simulink model "RegolazioneDinamicaSistemaNonLineare_mdl"  (Simulink 7.2)
settings: Solver=ode45  StartTime=0.0  StopTime=30  RelTol=1e-3
values from neighbouring files (symbols this model uses):
  b = 0.0575    [TSC150918ProvaMatlab.m]
  C1 = [1 -1 0 0]    [TSC150918ProvaMatlab.m]
  d = 2.5185    [TSC150918ProvaMatlab.m]
  g = 9.81    [TSC150918ProvaMatlab.m]
  j = 0.2156    [TSC150918ProvaMatlab.m]
  k = 200    [TSC150918ProvaMatlab.m]
  l = 0.5    [TSC150918ProvaMatlab.m]
  L = - acker(A',C1',Po)'    [TSC150918ProvaMatlab.m]
  m = 0.15    [TSC150918ProvaMatlab.m]
  taue = 0.2    [TSC150918ProvaMatlab.m]
  X0 = Xe + Dx0    [TSC150918ProvaMatlab.m]
undefined symbols (not defined in the file or in its folder): A, B, K
settings Model: Creator=lbiagiotti  LastModifiedBy=lbiagiotti

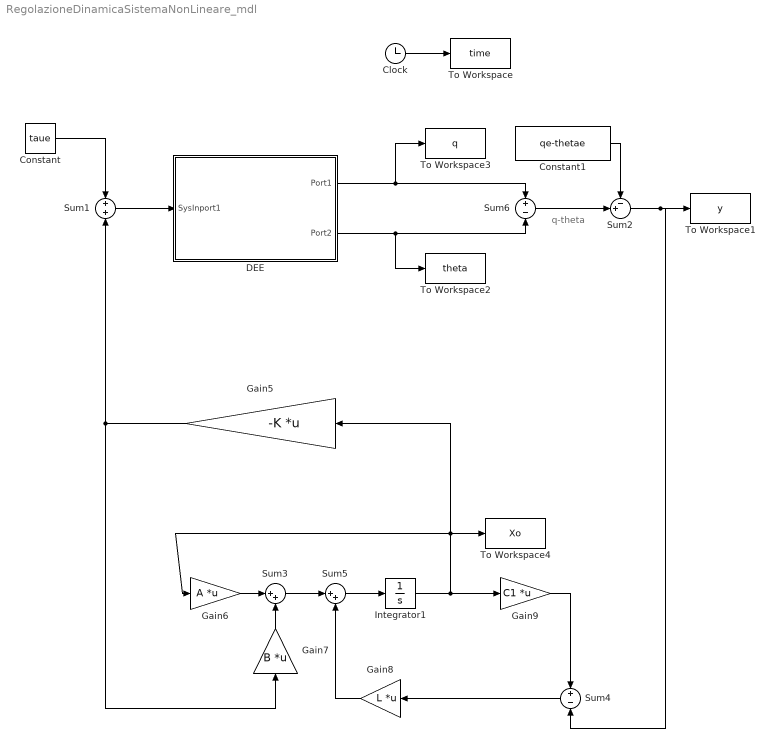
== system RegolazioneDinamicaSistemaNonLineare_mdl ==
  note: q-theta
  Clock : Clock
      settings: Decimation=10
  Constant : Constant  Value=taue  OutDataType=sfix(16)  OutScaling=2^0
  Constant1 : Constant  Value=qe-thetae  OutDataType=sfix(16)  OutScaling=2^0
  DEE : Subsystem
      settings: OpenFcn=diffeqed
      mask Type: Differential Equation Editor (DEE)
      mask Display: disp('Differential Equation\n Editor')
  Gain5 : Gain  Orientation=left  Gain=-K  Multiplication=Matrix(K*u)  ParameterDataType=sfix(16)  ParameterScaling=2^0  OutDataType=sfix(16)  OutScaling=2^0
  Gain6 : Gain  Gain=A  Multiplication=Matrix(K*u)  ParameterDataType=sfix(16)  ParameterScaling=2^0  OutDataType=sfix(16)  OutScaling=2^0
  Gain7 : Gain  Orientation=up  Gain=B  Multiplication=Matrix(K*u)  ParameterDataType=sfix(16)  ParameterScaling=2^0  OutDataType=sfix(16)  OutScaling=2^0
  Gain8 : Gain  Orientation=left  Gain=L  Multiplication=Matrix(K*u)  ParameterDataType=sfix(16)  ParameterScaling=2^0  OutDataType=sfix(16)  OutScaling=2^0
  Gain9 : Gain  Gain=C1  Multiplication=Matrix(K*u)  ParameterDataType=sfix(16)  ParameterScaling=2^0  OutDataType=sfix(16)  OutScaling=2^0
  Integrator1 : Integrator  InitialCondition=[0 0 0 0]
  Sum1 : Sum  OutDataType=sfix(16)  OutScaling=2^0
  Sum2 : Sum  Inputs=-+|  OutDataType=sfix(16)  OutScaling=2^0
  Sum3 : Sum  Inputs=|++  OutDataType=sfix(16)  OutScaling=2^0
  Sum4 : Sum  Orientation=left  Inputs=+-  OutDataType=sfix(16)  OutScaling=2^0
  Sum5 : Sum  Inputs=|++  OutDataType=sfix(16)  OutScaling=2^0
  Sum6 : Sum  Inputs=+-  OutDataType=sfix(16)  OutScaling=2^0
  To Workspace : ToWorkspace  VariableName=time  SampleTime=-1  SaveFormat=Array
  To Workspace1 : ToWorkspace  VariableName=y  SampleTime=-1  SaveFormat=Array
  To Workspace2 : ToWorkspace  VariableName=theta  SampleTime=-1  SaveFormat=Array
  To Workspace3 : ToWorkspace  VariableName=q  SampleTime=-1  SaveFormat=Array
  To Workspace4 : ToWorkspace  VariableName=Xo  SampleTime=-1  SaveFormat=Array
  wires:
  Clock/1 -> To Workspace/1
  Gain5/1 -> Gain7/1, Sum1/2
  Gain6/1 -> Sum3/1
  Integrator1/1 -> Gain9/1, Gain6/1, To Workspace4/1, Gain5/1
  Gain7/1 -> Sum3/2
  Sum4/1 -> Gain8/1
  Gain8/1 -> Sum5/2
  Sum3/1 -> Sum5/1
  Sum5/1 -> Integrator1/1
  Gain9/1 -> Sum4/1
  Sum1/1 -> DEE/1(SysInport1)
  Constant/1 -> Sum1/1
  Sum2/1 -> To Workspace1/1, Sum4/2
  Constant1/1 -> Sum2/1
  DEE/1(Port1) -> Sum6/1, To Workspace3/1
  DEE/2(Port2) -> Sum6/2, To Workspace2/1
  Sum6/1 -> Sum2/2

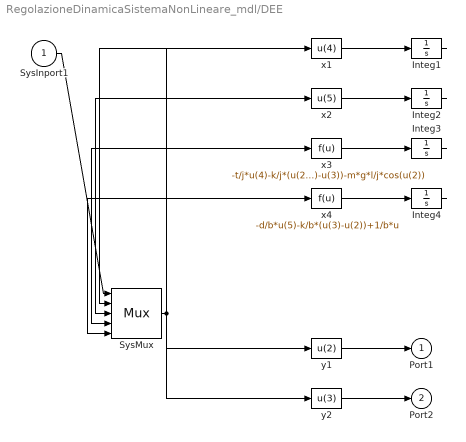
== system RegolazioneDinamicaSistemaNonLineare_mdl/DEE ==
  SysInport1 : Inport
  Integ1 : Integrator  InitialCondition=X0(1)
  Integ2 : Integrator  InitialCondition=X0(2)
  Integ3 : Integrator  InitialCondition=X0(3)
  Integ4 : Integrator  InitialCondition=X0(4)
  SysMux : Mux  Inputs=5
  x1 : Fcn  Expr=u(4)
  x2 : Fcn  Expr=u(5)
  x3 : Fcn  Expr=-t/j*u(4)-k/j*(u(2)-u(3))-m*g*l/j*cos(u(2))
  x4 : Fcn  Expr=-d/b*u(5)-k/b*(u(3)-u(2))+1/b*u
  y1 : Fcn  Expr=u(2)
  y2 : Fcn  Expr=u(3)
  Port1 : Outport
  Port2 : Outport  Port=2
  wires:
  SysInport1/1 -> SysMux/1
  SysMux/1 -> x1/1, x2/1, x3/1, x4/1, y1/1, y2/1
  x1/1 -> Integ1/1
  Integ1/1 -> SysMux/2
  x2/1 -> Integ2/1
  Integ2/1 -> SysMux/3
  x3/1 -> Integ3/1
  Integ3/1 -> SysMux/4
  x4/1 -> Integ4/1
  Integ4/1 -> SysMux/5
  y1/1 -> Port1/1
  y2/1 -> Port2/1
